simulink model "WithArrester"  (R2025a)
settings: Solver=ode23tb  StartTime=0.0  StopTime=.1  RelTol=1e-3  EnableMultiTasking=on
libraries: spsSeriesRLCBranchLib x6, spsGroundLib x4, spsControlledVoltageSourceLib x3, spsSurgeArresterLib x3, spsThreePhaseVIMeasurementLib x2, spsThreePhaseSourceLib x1, simulink x1, spsThreePhaseParallelRLCLoadLib x1, spsThreePhasePISectionLineLib x1, sps_lib x1
settings Model: Creator=Rodney Tan  LastModifiedBy=Sanny
settings SolverCC: AlgebraicLoopSolver=TrustRegion
settings DataIOCC: LimitDataPoints=on  SaveFormat=Array  ReturnWorkspaceOutputs=off
settings OptimizationCC: LifeSpan=inf
settings DebuggingCC: SolverPrmCheckMsg=warning  UnconnectedInputMsg=warning  UnconnectedOutputMsg=warning  UnconnectedLineMsg=warning  SFUnexpectedBacktrackingDiag=warning  SFNoUnconditionalDefaultTransitionDiag=warning  SFExecutionAtInitializationDiag=none  ArithmeticOperatorsInVariantConditions=warning
settings HardwareCC: ProdBitPerPointer=32.0  ProdBitPerSizeT=32.0  ProdBitPerPtrDiffT=32.0  ProdLargestAtomicFloat=None  ProdIntDivRoundTo=Undefined  ProdEndianess=Unspecified  ProdWordSize=32.0  ProdHWDeviceType=32-bit Generic
settings ModelReferenceCC: EnableRefExpFcnMdlSchedulingChecks=on  PropagateSignalLabelsOutOfModel=off
settings SFSimCC: SimUseLocalCustomCode=off  CustomCodeUndefinedFunction=UseInterfaceOnly
settings RTWCC: RTWUseLocalCustomCode=off  GPUComputeCapability=3.5
settings CodeAppCC: StateflowObjectComments=on
settings GRTTargetCC: TargetLangStandard=C89/C90 (ANSI)
settings ConfigComp: CovMetricSettings=dw  CovSaveCumulativeToWorkspaceVar=on  CovSaveSingleToWorkspaceVar=on  CovExternalEMLEnable=off  CovSFcnEnable=off
settings SimscapeCC: SimscapeNormalizeSystem=off

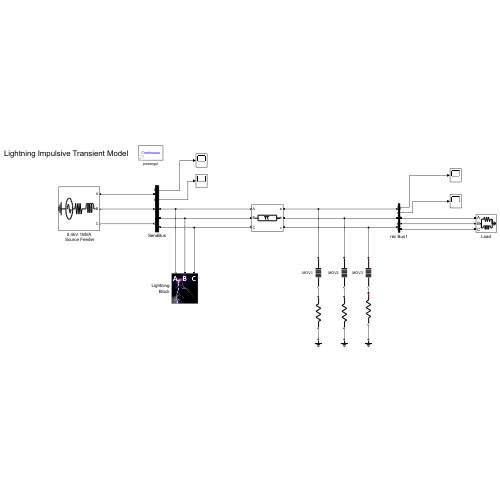
[thumbnail: Simulink's stored preview of the top-level diagram]
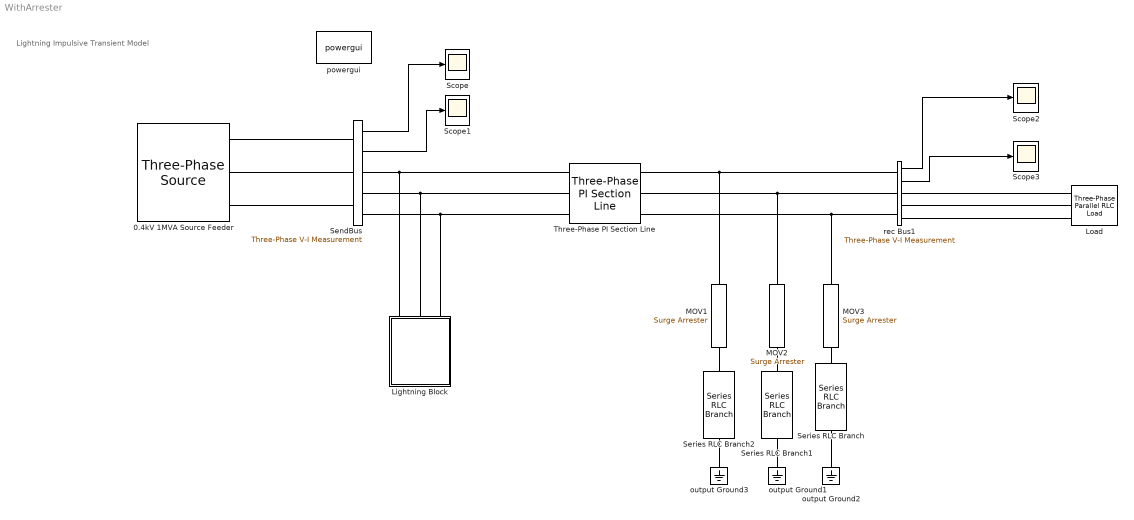
== system WithArrester ==
  note: Lightning Impulsive Transient Model
  0.4kV 1MVA Source Feeder : spsThreePhaseSourceLib/Three-Phase Source  InternalConnection=Yg  VoltagePhases=off  Voltage=0.4e3  PhaseAngle=0  Voltage_phases=[25e3 25e3 25e3]/sqrt(3)  PhaseAngles_phases=[0 -120 +120]  Frequency=50  NonIdealSource=on  SpecifyImpedance=on  Resistance=0.8929  Inductance=16.58e-3  ShortCircuitLevel=1e6  BaseVoltage=0.4e3  XRratio=7  BusType=swing  Pref=0  Qref=0  Prefabc=[10e3, 10e3, 10e3]  Qrefabc=[0, 0, 0]  Qmin=-inf  Qmax=inf
  Lightning Block : Subsystem  mask(Lightning Model){mag=100e3, t1=.055, R=1, L=1e-6}
      mask prompts: mag "Impulse Magnitude"; t1 "Impulse Start Time (s)"; R "Coupling Resistance (Ohms)"; L "Coupling Inductance (H)"
      mask help:
      | This lightning model simulate a 1.2/50us impulsive transient voltage defined by IEEE 1159.1 Standard. The impulsive transient is model by
      |
      | v = A*exp(-alpha*abs(t-t1))*u;
      |
      | where A is the impulse magnitude, t1 is the impulse start time, alpha is the damping factor of 14000 and u is the step function.
      mask DialogControl Container3 Prompt: Lightning Coupling
      mask Display: image('LightningBlock.jpg');
  Load : spsThreePhaseParallelRLCLoadLib/Three-Phase Parallel RLC Load  LConnTagsString=A|B|C  Configuration=Y (grounded)  NominalVoltage=0.4e3  Vabc=[1e3 1e3 1e3]  Vabcp=[1e3 1e3 1e3]  NominalFrequency=50  UnbalancedPower=off  ActivePower=10e3  InductivePower=100  CapacitivePower=0  Pabc=[10e3 9e3 11e3]  QLabc=[100 90 110]  QCabc=[100 90 110]  Pabcp=[10e3 9e3 11e3]  QLabcp=[100 90 110]  QCabcp=[100 90 110]  Measurements=None  LoadType=constant Z
  MOV1 : spsSurgeArresterLib/Surge Arrester  ProtectionVoltage=.18e3  Columns=10  ReferenceCurrent=500  Segment1=[.955 50]  Segment2=[1.0 25]  Segment3=[.9915 16.5]  Measurements=None  BreakLoop=off  UseDiscreteRobustSolver=on
      settings: AttributesFormatString=\n  LibrarySourceBlock=sps_lib/Passives/Surge Arrester
  MOV2 : spsSurgeArresterLib/Surge Arrester  ProtectionVoltage=.18e3  Columns=10  ReferenceCurrent=500  Segment1=[.955 50]  Segment2=[1.0 25]  Segment3=[.9915 16.5]  Measurements=None  BreakLoop=off  UseDiscreteRobustSolver=on
      settings: AttributesFormatString=\n  LibrarySourceBlock=sps_lib/Passives/Surge Arrester
  MOV3 : spsSurgeArresterLib/Surge Arrester  ProtectionVoltage=.18e3  Columns=10  ReferenceCurrent=500  Segment1=[.955 50]  Segment2=[1.0 25]  Segment3=[.9915 16.5]  Measurements=None  BreakLoop=off  UseDiscreteRobustSolver=on
      settings: AttributesFormatString=\n  LibrarySourceBlock=sps_lib/Passives/Surge Arrester
  Scope{,1..3} (4 alike) : Scope
      Scope settings: Title=Sending End Bus Voltage Profile  ShowGrid=off  ActiveDisplayYMinimum=-25226.28205  ActiveDisplayYMaximum=151040.12026  YLabel=Voltage (V)
      Scope1 settings: Title=Sending End Bus Current Profile  ShowGrid=off  ActiveDisplayYMinimum=-11708.72089  ActiveDisplayYMaximum=1655.21963  YLabel=Current (A)
      Scope2 settings: Title=Recieving End Bus Voltage Profile  ShowGrid=off  ActiveDisplayYMinimum=-182.01456538120124  ActiveDisplayYMaximum=189.61393404521641  YLabel=Voltage (V)  DataLoggingVariableName=ScopeData2
      Scope3 settings: Title=Recieving End Bus Current Profile  ShowGrid=off  ActiveDisplayYMinimum=-11.355164746020828  ActiveDisplayYMaximum=11.839411409521356  YLabel=Current (A)  DataLoggingVariableName=ScopeData3
  SendBus : spsThreePhaseVIMeasurementLib/Three-Phase V-I Measurement  VoltageMeasurement=phase-to-ground  SetLabelV=off  LabelV=Vabc  Vpu=off  VpuLL=off  CurrentMeasurement=yes  SetLabelI=off  LabelI=Iabc  Ipu=off  Pbase=100e6  Vbase=500e3  OutputType=Complex  PhasorSimulation=off  PSBequivalent=0
  Series RLC Branch : spsSeriesRLCBranchLib/Series RLC Branch  LConnTagsString=__new0  RConnTagsString=__new0  BranchType=R  Resistance=.001  Inductance=1e-3  SetiL0=off  InitialCurrent=0  Capacitance=1e-6  Setx0=off  InitialVoltage=0  Measurements=None
  Series RLC Branch1 : spsSeriesRLCBranchLib/Series RLC Branch  LConnTagsString=__new0  RConnTagsString=__new0  BranchType=R  Resistance=.001  Inductance=1e-3  SetiL0=off  InitialCurrent=0  Capacitance=1e-6  Setx0=off  InitialVoltage=0  Measurements=None
  Series RLC Branch2 : spsSeriesRLCBranchLib/Series RLC Branch  LConnTagsString=__new0  RConnTagsString=__new0  BranchType=R  Resistance=.001  Inductance=1e-3  SetiL0=off  InitialCurrent=0  Capacitance=1e-6  Setx0=off  InitialVoltage=0  Measurements=None
  Three-Phase PI Section Line : spsThreePhasePISectionLineLib/Three-Phase PI Section Line  LConnTagsString=a|b|c  RConnTagsString=A|B|C  Length=100  Frequency=60  Resistances=[ 0.01273 0.3864]  Inductances="[ 0.9337e-3  4.1264e-3]"  Capacitances=[12.74e-9 7.751e-9]
  output Ground1 : spsGroundLib/Ground  LConnTagsString=a
  output Ground2 : spsGroundLib/Ground  LConnTagsString=a
  output Ground3 : spsGroundLib/Ground  LConnTagsString=a
  powergui : sps_lib/powergui  Priority=1  SimulationMode=Continuous  SampleTime=50e-6  frequency=60  Iterations=50  frequencyindice=0  Pbase=100e6  ErrMax=1e-4  UnitsV=kV  UnitsW=MW  buscounter=0  FunctionMessages=off  echomessages=off  EnableUseOfTLC=off  CurrentSourceSwitches=on  DisableSnubberDevices=off  DisableRonSwitches=off  DisableVfSwitches=off  DisplayEquations=off  AutomaticDiscreteSolvers=off  SolverType=Tustin  Interpol=off  ExternalGateDelay=off  methode=off  Ts=0  x0status=blocks  SPID=off  SwTol=0  HookPort=off  NonlinearTolerance=1e-4  nMaxIteration=100  ContinueOnMaxIteration=off  RestoreLinks=warning  ResistiveCurrentMeasurement=off  Frange=[0:2:500]  Ylog=off  Xlog=on  ShowGrid=off  save=off  variable=ZData  structure=0  ZoomFFT=off  StartTime=0.0  cycles=1  DisplayStyle=1  fundamental=60  FreqAxis=off  MaxFrequency=1000  frequencyindicesteady=1  RmsSteady=1  display=off
  rec Bus1 : spsThreePhaseVIMeasurementLib/Three-Phase V-I Measurement  VoltageMeasurement=phase-to-ground  SetLabelV=off  LabelV=Vabc  Vpu=off  VpuLL=off  CurrentMeasurement=yes  SetLabelI=off  LabelI=Iabc  Ipu=off  Pbase=100e6  Vbase=500e3  OutputType=Complex  PhasorSimulation=off  PSBequivalent=0
  wires:
  SendBus/1 -> Scope/1
  SendBus/2 -> Scope1/1
  rec Bus1/1 -> Scope2/1
  rec Bus1/2 -> Scope3/1
  connections:
  0.4kV 1MVA Source Feeder/RConn2 -- SendBus/LConn2
  0.4kV 1MVA Source Feeder/RConn3 -- SendBus/LConn3
  0.4kV 1MVA Source Feeder/RConn1 -- SendBus/LConn1
  Series RLC Branch/RConn1 -- output Ground2/LConn1
  MOV3/RConn1 -- Series RLC Branch/LConn1
  Load/LConn3 -- rec Bus1/RConn3
  rec Bus1/RConn2 -- Load/LConn2
  rec Bus1/RConn1 -- Load/LConn1
  SendBus/RConn3 -- Three-Phase PI Section Line/LConn3 -- Lightning Block/LConn3
  Lightning Block/LConn2 -- Three-Phase PI Section Line/LConn2 -- SendBus/RConn2
  Lightning Block/LConn1 -- Three-Phase PI Section Line/LConn1 -- SendBus/RConn1
  Three-Phase PI Section Line/RConn3 -- MOV3/LConn1 -- rec Bus1/LConn3
  Three-Phase PI Section Line/RConn1 -- MOV1/LConn1 -- rec Bus1/LConn1
  Three-Phase PI Section Line/RConn2 -- MOV2/LConn1 -- rec Bus1/LConn2
  output Ground1/LConn1 -- Series RLC Branch1/RConn1
  output Ground3/LConn1 -- Series RLC Branch2/RConn1
  MOV2/RConn1 -- Series RLC Branch1/LConn1
  MOV1/RConn1 -- Series RLC Branch2/LConn1

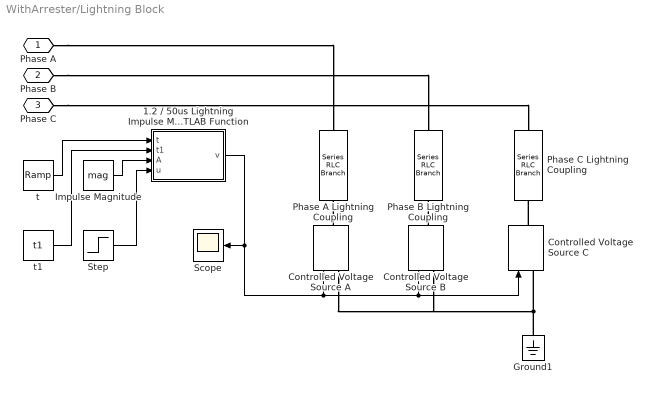
== system WithArrester/Lightning Block ==
  1.2 / 50us Lightning Impulse MATLAB Function : MATLAB Function  TreatAsAtomicUnit=on
  Controlled Voltage Source C : spsControlledVoltageSourceLib/Controlled Voltage Source  Initialize=on  Source_Type=DC  Amplitude=0  Phase=0  Frequency=0  Measurements=None
  Controlled Voltage Source A : spsControlledVoltageSourceLib/Controlled Voltage Source  Initialize=on  Source_Type=DC  Amplitude=0  Phase=0  Frequency=0  Measurements=None
  Controlled Voltage Source B : spsControlledVoltageSourceLib/Controlled Voltage Source  Initialize=on  Source_Type=DC  Amplitude=0  Phase=0  Frequency=0  Measurements=None
  Ground1 : spsGroundLib/Ground  LConnTagsString=a
  Impulse Magnitude : Constant  Value=mag
  Phase A Lightning Coupling : spsSeriesRLCBranchLib/Series RLC Branch  LConnTagsString=__new0  RConnTagsString=__new0  BranchType=RL  Resistance=R  Inductance=L  SetiL0=off  InitialCurrent=0  Capacitance=1e-6  Setx0=off  InitialVoltage=0  Measurements=None
  Phase B Lightning Coupling : spsSeriesRLCBranchLib/Series RLC Branch  LConnTagsString=__new0  RConnTagsString=__new0  BranchType=RL  Resistance=R  Inductance=L  SetiL0=off  InitialCurrent=0  Capacitance=1e-6  Setx0=off  InitialVoltage=0  Measurements=None
  Phase C Lightning Coupling : spsSeriesRLCBranchLib/Series RLC Branch  LConnTagsString=__new0  RConnTagsString=__new0  BranchType=RL  Resistance=R  Inductance=L  SetiL0=off  InitialCurrent=0  Capacitance=1e-6  Setx0=off  InitialVoltage=0  Measurements=None
  Scope : Scope
      settings: SampleTime=1/1e6  DataLoggingSaveFormat=Array
  Step : Step  Time=t1  SampleTime=0
  t : simulink/Sources/Ramp  slope=1  start=0  InitialOutput=0
  t1 : Constant  Value=t1
  Phase A : PMIOPort  Side=Left
  Phase B : PMIOPort  Port=2  Side=Left
  Phase C : PMIOPort  Port=3  Side=Left
  wires:
  1.2 / 50us Lightning Impulse MATLAB Function/1(v) -> Scope/1, Controlled Voltage Source A/1, Controlled Voltage Source C/1, Controlled Voltage Source B/1
  t/1 -> 1.2 / 50us Lightning Impulse MATLAB Function/1(t)
  t1/1 -> 1.2 / 50us Lightning Impulse MATLAB Function/2(t1)
  Impulse Magnitude/1 -> 1.2 / 50us Lightning Impulse MATLAB Function/3(A)
  Step/1 -> 1.2 / 50us Lightning Impulse MATLAB Function/4(u)
  connections:
  Ground1/LConn1 -- Controlled Voltage Source A/LConn1 -- Controlled Voltage Source B/LConn1 -- Controlled Voltage Source C/LConn1
  Controlled Voltage Source C/RConn1 -- Phase C Lightning Coupling/RConn1
  Controlled Voltage Source A/RConn1 -- Phase A Lightning Coupling/RConn1
  Phase A/RConn1 -- Phase A Lightning Coupling/LConn1
  Phase B/RConn1 -- Phase B Lightning Coupling/LConn1
  Controlled Voltage Source B/RConn1 -- Phase B Lightning Coupling/RConn1
  Phase C/RConn1 -- Phase C Lightning Coupling/LConn1

== matlab function WithArrester/Lightning Block/1.2 // 50us Lightning Impulse MATLAB Function ==
  data: t input; t1 input; A input; v output; u input
function v = fcn(t,t1,A,u)
alpha=14000;
v = A*exp(-alpha*abs(t-t1))*u;
